simulink model "CompFilterForAngle"  (R2021a)
settings: Solver=VariableStepAuto  StartTime=0.0  StopTime=10.0  RelTol=1e-3
undefined symbols (not defined in the file or in its folder): dt, ts
settings Model: Creator=tocay  LastModifiedBy=tocay

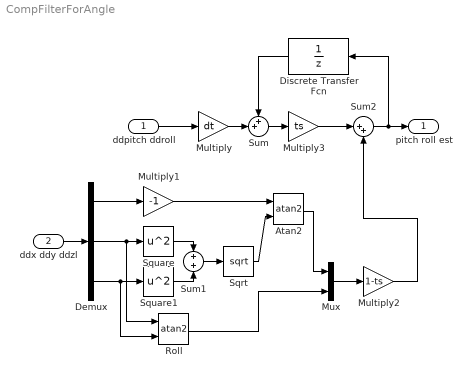
== system CompFilterForAngle ==
  ddpitch ddroll : Inport
  ddx ddy ddzl : Inport  Port=2
  Atan2 : Trigonometry  Operator=atan2
  Demux : Demux  Outputs=3
  Discrete Transfer Fcn : DiscreteTransferFcn  Denominator=[1 0]
  Multiply : Gain  Gain=dt
  Multiply1 : Gain  Gain=-1
  Multiply2 : Gain  Gain=1-ts
  Multiply3 : Gain  Gain=ts
  Mux : Mux  Inputs=2
  Roll : Trigonometry  Operator=atan2
  Sqrt : Sqrt  SaturateOnIntegerOverflow=on
  Square : Math  Operator=square  SaturateOnIntegerOverflow=on
  Square1 : Math  Operator=square  SaturateOnIntegerOverflow=on
  Sum : Sum  Inputs=++|
  Sum1 : Sum
  Sum2 : Sum  Inputs=|++
  pitch roll est : Outport
  wires:
  ddpitch ddroll/1 -> Multiply/1
  ddx ddy ddzl/1 -> Demux/1
  Demux/2 -> Roll/1, Square/1
  Demux/3 -> Roll/2, Square1/1
  Demux/1 -> Multiply1/1
  Multiply1/1 -> Atan2/1
  Square/1 -> Sum1/1
  Square1/1 -> Sum1/2
  Sum1/1 -> Sqrt/1
  Sqrt/1 -> Atan2/2
  Atan2/1 -> Mux/1
  Roll/1 -> Mux/2
  Multiply/1 -> Sum/2
  Discrete Transfer Fcn/1 -> Sum/1
  Sum/1 -> Multiply3/1
  Mux/1 -> Multiply2/1
  Multiply3/1 -> Sum2/1
  Multiply2/1 -> Sum2/2
  Sum2/1 -> Discrete Transfer Fcn/1, pitch roll est/1
